simulink model "LFC_3area_fastLoadActor"  (R2021b)
settings: Solver=FixedStepAuto  StartTime=0.0  StopTime=350  FixedStep=0.01  RelTol=1e-3
undefined symbols (not defined in the file or in its folder): sigbuilder_block
libraries: deeplib x3
settings Model: Creator=abc19  LastModifiedBy=abc19
settings SolverCC: AlgebraicLoopSolver=TrustRegion
settings DebuggingCC: SFMachineParentedDataDiag=warning
settings SFSimCC: SimTargetLang=C++

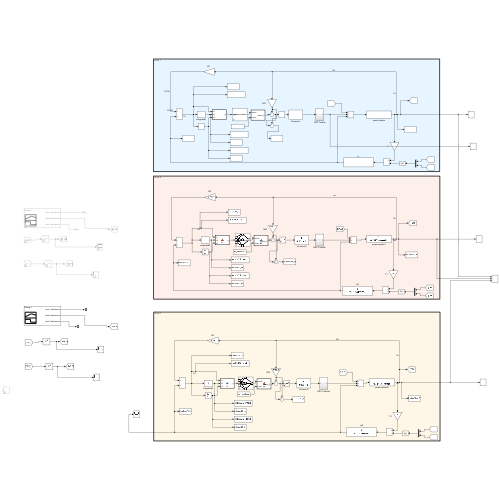
[thumbnail: Simulink's stored preview of the top-level diagram]
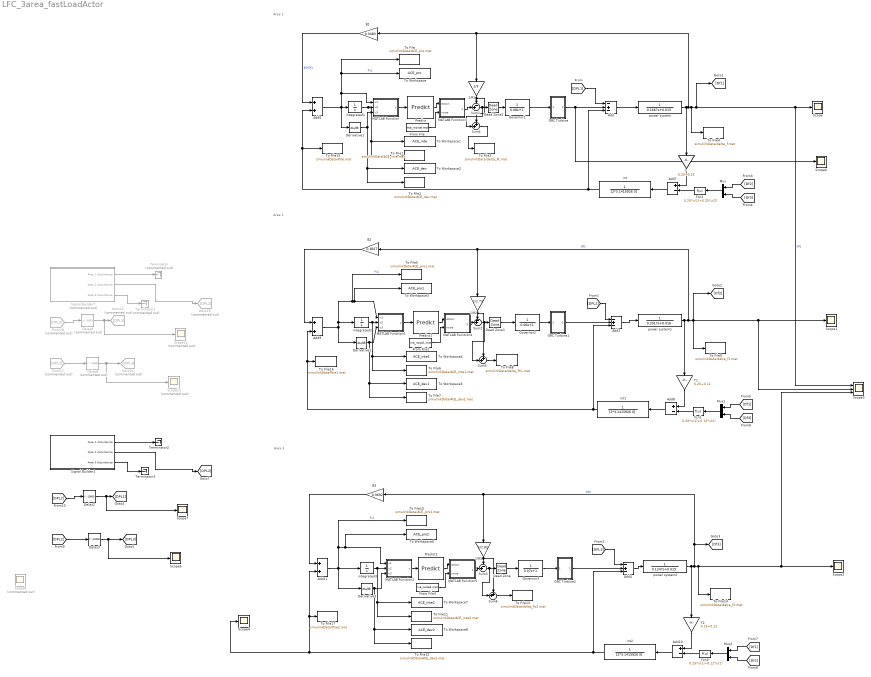
== system LFC_3area_fastLoadActor ==
  note: Area 1
  note: Area 3
  note: Area 2
  1/R1 : Gain  Gain=1/3
  1/R2 : Gain  Gain=1/2.73
  1/R3 : Gain  Gain=1/2.82
  Add : Sum  Inputs=-+-
  Add10 : Sum  Inputs=+-
  Add11 : Sum
  Add2 : Sum  Inputs=-+-
  Add4 : Sum  Inputs=-+-
  Add6 : Sum
  Add7 : Sum  Inputs=+-
  Add8 : Sum  Inputs=+-
  Add9 : Sum
  B1 : Gain  Gain=0.3483
  B2 : Gain  Gain=0.3827
  B3 : Gain  Gain=0.3692
  Dead Zone : DeadZone  LowerValue=-0.00638  UpperValue=0.00638  SaturateOnIntegerOverflow=on
  Dead Zone1 : DeadZone  LowerValue=-0.00659  UpperValue=0.00659  SaturateOnIntegerOverflow=on
  Dead Zone2 : DeadZone  LowerValue=-0.006  UpperValue=0.006  SaturateOnIntegerOverflow=on
  Delay2 : Delay  DelayLength=10000  InitialCondition=0
  Delay3 : Delay  DelayLength=20000  InitialCondition=0
  Delay8 : Delay  Commented=on  DelayLength=5000  InitialCondition=0
  Delay9 : Delay  Commented=on  DelayLength=10000  InitialCondition=0
  Derivative1 : Derivative
  Derivative2 : Derivative
  Derivative3 : Derivative
  Fcn1 : Fcn  Expr=0.20*u(1)+0.12*u(2)
  Fcn2 : Fcn  Expr=0.20*u(1)+0.25*u(2)
  Fcn3 : Fcn  Expr=0.25*u(1)+0.12*u(2)
  From File : FromFile  FileName=ma_noise.mat  SampleTime=0
  From File1 : FromFile  FileName=ma_noise1.mat  SampleTime=0
  From File3 : FromFile  FileName=ma_noise2.mat  SampleTime=0
  From17 : From  Commented=on  GotoTag=DPL2
  From18 : From  Commented=on  GotoTag=DPL2
  GRC Turbine : Subsystem
  GRC Turbine1 : Subsystem
  GRC Turbine2 : Subsystem
  Goto22 : Goto  Commented=on  GotoTag=DPL1
  Goto23 : Goto  Commented=on  GotoTag=DPL3
  Goto25 : Goto  Commented=on  GotoTag=DPL2
  Governor1 : TransferFcn  Denominator=[0.08 1]
  Governor2 : TransferFcn  Denominator=[0.06 1]
  Governor3 : TransferFcn  Denominator=[0.07 1]
  MATLAB Function : MATLAB Function  TreatAsAtomicUnit=on  SystemSampleTime=0.01
  MATLAB Function1 : MATLAB Function  TreatAsAtomicUnit=on  SystemSampleTime=0.01
  MATLAB Function2 : MATLAB Function  TreatAsAtomicUnit=on  SystemSampleTime=0.01
  MATLAB Function3 : MATLAB Function  TreatAsAtomicUnit=on  SystemSampleTime=0.01
  MATLAB Function4 : MATLAB Function  TreatAsAtomicUnit=on  SystemSampleTime=0.01
  MATLAB Function5 : MATLAB Function  TreatAsAtomicUnit=on  SystemSampleTime=0.01
  Mux : Mux  Inputs=2
  Mux1 : Mux  Inputs=2
  Mux2 : Mux  Inputs=2
  Predict : deeplib/Predict  Network=Network from MAT-file  NetworkFunction=squeezenet  NetworkFilePath=aaa.mat  MiniBatchSize=1  InputDataFormats={ '', '' }  Predictions=on  Activations={}  ForceInterpretedSim=off  EnableDLNetwork=on
      settings: SourceProductBaseCode=NN
  Predict1 : deeplib/Predict  Network=Network from MAT-file  NetworkFunction=squeezenet  NetworkFilePath=bbb.mat  MiniBatchSize=1  InputDataFormats={ '', '' }  Predictions=on  Activations={}  ForceInterpretedSim=off  EnableDLNetwork=on
      settings: SourceProductBaseCode=NN
  Predict2 : deeplib/Predict  Network=Network from MAT-file  NetworkFunction=squeezenet  NetworkFilePath=ccc.mat  MiniBatchSize=1  InputDataFormats={ '', '' }  Predictions=on  Activations={}  ForceInterpretedSim=off  EnableDLNetwork=on
      settings: SourceProductBaseCode=NN
  Scope{,1..2,4..7} (7 alike) : Scope
  Scope13 : Scope  Commented=on
  Scope14 : Scope  Commented=on
  Scope3 : Scope  NumInputPorts=3
  Scope8 : Scope  Commented=on
  Signal Builder1 : Subsystem  Tag=STV Subsys  LoadFcn=sigbuilder_block('load');  StartFcn=sigbuilder_block('start');  StopFcn=sigbuilder_block('stop');  ClipboardFcn=sigbuilder_block('clipboard');  mask(Sigbuilder block){tuvar=[0:10]}
      mask help: Simulink:masks:SigbuilderBlock_MD
      mask init:
      | if ~strcmp(get_param(bdroot(gcbh),'SimulationStatus'),'stopped') tuvar = sigbuilder_block('maskInit'); end
      settings: CopyFcn=sigbuilder_block('copy');  DeleteFcn=sigbuilder_block('delete');  ModelCloseFcn=sigbuilder_block('modelClose');  PreSaveFcn=sigbuilder_block('preSave');  PauseFcn=sigbuilder_block('pause');  ContinueFcn=sigbuilder_block('continue');  NameChangeFcn=sigbuilder_block('namechange');  OpenFcn=sigbuilder_block('open',[259.2 170.4 1141.2 408.6 ]);  CloseFcn=sigbuilder_block('close');
      mask Display: plot(0, 0, 100, 100,[2, 2, 32, 32, 2], [68, 8, 8, 68, 68],[32, 2], [38, 38], [32, 19, 2],[53, 60, 44], [32, 17, 17, 2],[16, 16, 31, 31]);txt = getActiveGroup(gcbh);text(2, 100, txt,'verticalAlignment', 'top');
  Signal Builder7 : Subsystem  Tag=STV Subsys  Commented=on  LoadFcn=sigbuilder_block('load');  StartFcn=sigbuilder_block('start');  StopFcn=sigbuilder_block('stop');  ClipboardFcn=sigbuilder_block('clipboard');  mask(Sigbuilder block){tuvar=[0:10]}
      mask help: Simulink:masks:SigbuilderBlock_MD
      mask init:
      | if ~strcmp(get_param(bdroot(gcbh),'SimulationStatus'),'stopped') tuvar = sigbuilder_block('maskInit'); end
      settings: CopyFcn=sigbuilder_block('copy');  DeleteFcn=sigbuilder_block('delete');  ModelCloseFcn=sigbuilder_block('modelClose');  PreSaveFcn=sigbuilder_block('preSave');  PauseFcn=sigbuilder_block('pause');  ContinueFcn=sigbuilder_block('continue');  NameChangeFcn=sigbuilder_block('namechange');  OpenFcn=sigbuilder_block('open',[69 85.8 1141.2 485.4 ]);  CloseFcn=sigbuilder_block('close');
      mask Display: plot(0, 0, 100, 100,[2, 2, 32, 32, 2], [68, 8, 8, 68, 68],[32, 2], [38, 38], [32, 19, 2],[53, 60, 44], [32, 17, 17, 2],[16, 16, 31, 31]);txt = getActiveGroup(gcbh);text(2, 100, txt,'verticalAlignment', 'top');
  Sum1 : Sum  Inputs=-+|
  Sum2 : Sum  Inputs=-+|
  Sum3 : Sum  Inputs=-+|
  Sum4 : Sum  Inputs=++|
  Sum5 : Sum  Inputs=++|
  Sum6 : Sum  Inputs=++|
  T : Gain  Gain=0.20+0.25
  T1 : Gain  Gain=0.20+0.12
  T2 : Gain  Gain=0.25+0.12
  Terminator : Terminator  Commented=on
  Terminator1 : Terminator  Commented=on
  Terminator2 : Terminator
  Terminator3 : Terminator
  To File : ToFile  Filename=simulinkData/ACE_pro.mat  SampleTime=0.01
  To File1 : ToFile  Filename=simulinkData/ACE_inte.mat  SampleTime=0.01
  To File10 : ToFile  Filename=simulinkData/ACE_pro2.mat  SampleTime=0.01
  To File11 : ToFile  Filename=simulinkData/ACE_inte2.mat  SampleTime=0.01
  To File12 : ToFile  Filename=simulinkData/ACE_dev2.mat  SampleTime=0.01
  To File13 : ToFile  Filename=simulinkData/delta_Pc2.mat  SampleTime=0.01
  To File14 : ToFile  Filename=simulinkData/delta_f2.mat  SampleTime=0.01
  To File15 : ToFile  Filename=simulinkData/Ptie.mat  SampleTime=0.01
  To File16 : ToFile  Filename=simulinkData/Ptie1.mat  SampleTime=0.01
  To File17 : ToFile  Filename=simulinkData/Ptie2.mat  SampleTime=0.01
  To File2 : ToFile  Filename=simulinkData/ACE_dev.mat  SampleTime=0.01
  To File3 : ToFile  Filename=simulinkData/delta_Pc.mat  SampleTime=0.01
  To File4 : ToFile  Filename=simulinkData/delta_f.mat  SampleTime=0.01
  To File5 : ToFile  Filename=simulinkData/ACE_pro1.mat  SampleTime=0.01
  To File6 : ToFile  Filename=simulinkData/ACE_inte1.mat  SampleTime=0.01
  To File7 : ToFile  Filename=simulinkData/ACE_dev1.mat  SampleTime=0.01
  To File8 : ToFile  Filename=simulinkData/delta_Pc1.mat  SampleTime=0.01
  To File9 : ToFile  Filename=simulinkData/delta_f1.mat  SampleTime=0.01
  To Workspace : ToWorkspace  VariableName=ACE_pro  SaveFormat=Timeseries  SampleTime=0.01
  To Workspace1 : ToWorkspace  VariableName=ACE_inte  SaveFormat=Timeseries  SampleTime=0.01
  To Workspace2 : ToWorkspace  VariableName=ACE_dev  SaveFormat=Timeseries  SampleTime=0.01
  To Workspace3 : ToWorkspace  VariableName=ACE_pro1  SaveFormat=Timeseries  SampleTime=0.01
  To Workspace4 : ToWorkspace  VariableName=ACE_inte1  SaveFormat=Timeseries  SampleTime=0.01
  To Workspace5 : ToWorkspace  VariableName=ACE_dev1  SaveFormat=Timeseries  SampleTime=0.01
  To Workspace6 : ToWorkspace  VariableName=ACE_pro2  SaveFormat=Timeseries  SampleTime=0.01
  To Workspace7 : ToWorkspace  VariableName=ACE_inte2  SaveFormat=Timeseries  SampleTime=0.01
  To Workspace8 : ToWorkspace  VariableName=ACE_dev2  SaveFormat=Timeseries  SampleTime=0.01
  int : TransferFcn  Denominator=[2*3.1415926 0]
  int1 : TransferFcn  Denominator=[2*3.1415926 0]
  int2 : TransferFcn  Denominator=[2*3.1415926 0]
  integrated1 : TransferFcn  Denominator=[1 0]
  integrated2 : TransferFcn  Denominator=[1 0]
  integrated3 : TransferFcn  Denominator=[1 0]
  power system : TransferFcn  Denominator=[0.1667 0.015]
  power system1 : TransferFcn  Denominator=[0.2017 0.016]
  power system2 : TransferFcn  Denominator=[0.1247 0.015]
  wires:
  [DPL1] -> Add/1
  power system/1 -> To File4/1, [Df1], Scope3/1, Scope/1, B1/1, 1/R1/1, T/1  "Df1"
  GRC Turbine/1(Out1) -> Scope6/1, Add/2
  Add/1 -> power system/1
  B1/1 -> Add6/1  "B1*Df1"
  1/R1/1 -> Sum4/1, Sum1/1
  Governor1/1 -> GRC Turbine/1(In1)
  Sum1/1 -> Sum4/2, Dead Zone2/1
  Derivative1/1 -> To File2/1, To Workspace2/1, MATLAB Function/3(u3)
  integrated1/1 -> To File1/1, To Workspace1/1, MATLAB Function/2(u2)
  Add2/1 -> power system1/1
  Sum2/1 -> Sum5/2, Dead Zone1/1
  1/R2/1 -> Sum5/1, Sum2/1
  Governor2/1 -> GRC Turbine1/1(In1)
  GRC Turbine1/1(Out1) -> Add2/2
  [DPL2] -> Add2/1
  Add4/1 -> power system2/1
  Sum3/1 -> Sum6/2, Dead Zone/1
  1/R3/1 -> Sum6/1, Sum3/1
  Governor3/1 -> GRC Turbine2/1(In1)
  GRC Turbine2/1(Out1) -> Add4/2
  [DPL3] -> Add4/1
  int/1 -> Add6/2, To File15/1, Add/3
  Add6/1 -> Derivative1/1, To Workspace/1, To File/1, MATLAB Function/1(u1), integrated1/1  "Pc1"
  Add7/1 -> int/1
  T/1 -> Add7/1
  Fcn2/1 -> Add7/2
  Mux/1 -> Fcn2/1
  [Df2] -> Mux/1
  [Df3] -> Mux/2
  [Df1] -> Mux1/1
  [Df3] -> Mux1/2
  Mux1/1 -> Fcn1/1
  power system1/1 -> To File9/1, [Df2], Scope3/2, Scope1/1, B2/1, 1/R2/1, T1/1  "Df2"
  T1/1 -> Add8/1
  int1/1 -> To File16/1, Add9/2, Add2/3
  Add8/1 -> int1/1
  Fcn1/1 -> Add8/2
  B2/1 -> Add9/1
  [Df1] -> Mux2/1
  [Df2] -> Mux2/2
  Mux2/1 -> Fcn3/1
  power system2/1 -> [Df3], B3/1, 1/R3/1, To File14/1, Scope3/3, Scope2/1, T2/1  "Df3"
  T2/1 -> Add10/1
  int2/1 -> Scope4/1, To File17/1, Add11/2, Add4/3
  Add10/1 -> int2/1
  Fcn3/1 -> Add10/2
  B3/1 -> Add11/1
  Dead Zone/1 -> Governor3/1
  Dead Zone1/1 -> Governor2/1
  Dead Zone2/1 -> Governor1/1
  MATLAB Function/1(y) -> Predict/1
  MATLAB Function3/1(action_2) -> Sum1/2
  Predict/1 -> MATLAB Function3/1(action)
  Predict1/1 -> MATLAB Function4/1(action)
  integrated2/1 -> To File6/1, To Workspace4/1, MATLAB Function1/2(u2)
  MATLAB Function4/1(action_2) -> Sum2/2
  Derivative2/1 -> MATLAB Function1/3(u3), To File7/1, To Workspace5/1
  MATLAB Function1/1(y) -> Predict1/1
  Add9/1 -> Derivative2/1, MATLAB Function1/1(u1), To Workspace3/1, To File5/1, integrated2/1  "Pc1"
  Predict2/1 -> MATLAB Function5/1(action)
  integrated3/1 -> MATLAB Function2/2(u2), To File11/1, To Workspace7/1
  MATLAB Function5/1(action_2) -> Sum3/2
  Derivative3/1 -> MATLAB Function2/3(u3), To File12/1, To Workspace8/1
  MATLAB Function2/1(y) -> Predict2/1
  Add11/1 -> To File10/1, MATLAB Function2/1(u1), To Workspace6/1, Derivative3/1, integrated3/1  "Pc1"
  Sum4/1 -> To File3/1
  Sum5/1 -> To File8/1
  Sum6/1 -> To File13/1
  Signal Builder7/2(Area 2 disturbance) -> Goto25/1
  Delay8/1 -> Scope14/1, Goto22/1
  From17/1 -> Delay9/1
  Delay9/1 -> Goto23/1, Scope13/1
  From18/1 -> Delay8/1
  From File/1 -> MATLAB Function3/2(noise)
  From File1/1 -> MATLAB Function4/2(noise)
  From File3/1 -> MATLAB Function5/2(noise)
  Signal Builder7/1(Area 1 disturbance) -> Terminator/1
  Signal Builder7/3(Area 3 disturbance) -> Terminator1/1
  Signal Builder1/3(Area 3 disturbance) -> Terminator3/1
  Delay3/1 -> Scope5/1, [DPL3]
  Signal Builder1/2(Area 2 disturbance) -> [DPL2]
  [DPL2] -> Delay2/1
  [DPL2] -> Delay3/1
  Signal Builder1/1(Area 1 disturbance) -> Terminator2/1
  Delay2/1 -> [DPL1], Scope7/1

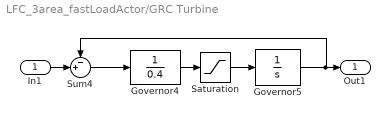
== system LFC_3area_fastLoadActor/GRC Turbine ==
  In1 : Inport
  Governor4 : TransferFcn  Denominator=[0.4]
  Governor5 : TransferFcn  Denominator=[1 0]
  Saturation : Saturate  UpperLimit=0.0017  LowerLimit=-0.0017
  Sum4 : Sum  Inputs=-+|
  Out1 : Outport
  wires:
  Governor5/1 -> Sum4/1, Out1/1
  Governor4/1 -> Saturation/1
  Sum4/1 -> Governor4/1
  Saturation/1 -> Governor5/1
  In1/1 -> Sum4/2

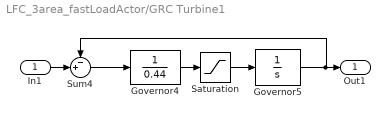
== system LFC_3area_fastLoadActor/GRC Turbine1 ==
  In1 : Inport
  Governor4 : TransferFcn  Denominator=[0.44]
  Governor5 : TransferFcn  Denominator=[1 0]
  Saturation : Saturate  UpperLimit=0.0017  LowerLimit=-0.0017
  Sum4 : Sum  Inputs=-+|
  Out1 : Outport
  wires:
  Governor5/1 -> Sum4/1, Out1/1
  Governor4/1 -> Saturation/1
  Sum4/1 -> Governor4/1
  Saturation/1 -> Governor5/1
  In1/1 -> Sum4/2

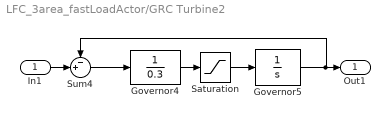
== system LFC_3area_fastLoadActor/GRC Turbine2 ==
  In1 : Inport
  Governor4 : TransferFcn  Denominator=[0.3]
  Governor5 : TransferFcn  Denominator=[1 0]
  Saturation : Saturate  UpperLimit=0.0017  LowerLimit=-0.0017
  Sum4 : Sum  Inputs=-+|
  Out1 : Outport
  wires:
  Governor5/1 -> Sum4/1, Out1/1
  Governor4/1 -> Saturation/1
  Sum4/1 -> Governor4/1
  Saturation/1 -> Governor5/1
  In1/1 -> Sum4/2

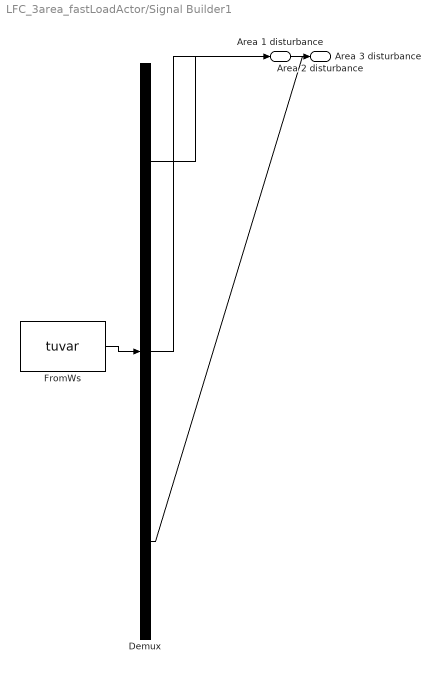
== system LFC_3area_fastLoadActor/Signal Builder1 ==
  Demux : Demux  Tag=STV Demux  Outputs=3
      settings: DisplayOption=none
  FromWs : FromWorkspace  Tag=STV FromWs  VariableName=tuvar
      SigBuilderData=|
      | common.afterFinalStr = 'Extrapolate'
      | common.sampleTime = 0
      | dataSet.timeRange = [0 400]
      | dataSet.name = 'Group 1'
      | sbobj.Groups.Name = 'Group 1'
      | sbobj.Groups.Signals(1).Name = 'Area 1 disturbance'
      | sbobj.Groups.Signals(1).XData = [0 30 30 60 60 400]
      | sbobj.Groups.Signals(1).YData = [0.01 0.01 -0.01 -0.01 0.01 0.01]
      | sbobj.Groups.Signals(2).Name = 'Area 2 disturbance'
      | sbobj.Groups.Signals(2).XData = [0 50 50 100 100 400]
      | sbobj.Groups.Signals(2).YData = [0 0 0.01 0.01 0 0]
      | sbobj.Groups.Signals(3).Name = 'Area 3 disturbance'
      | sbobj.Groups.Signals(3).XData = [0 400]
      | sbobj.Groups.Signals(3).YData = [0 0]
      | sbobj.Groups.TimeRange = [0 400]
  Area 1 disturbance : Outport  Tag=STV Outport
  Area 2 disturbance : Outport  Tag=STV Outport  Port=2
  Area 3 disturbance : Outport  Tag=STV Outport  Port=3
  wires:
  Demux/1 -> Area 1 disturbance/1
  FromWs/1 -> Demux/1
  Demux/2 -> Area 2 disturbance/1
  Demux/3 -> Area 3 disturbance/1

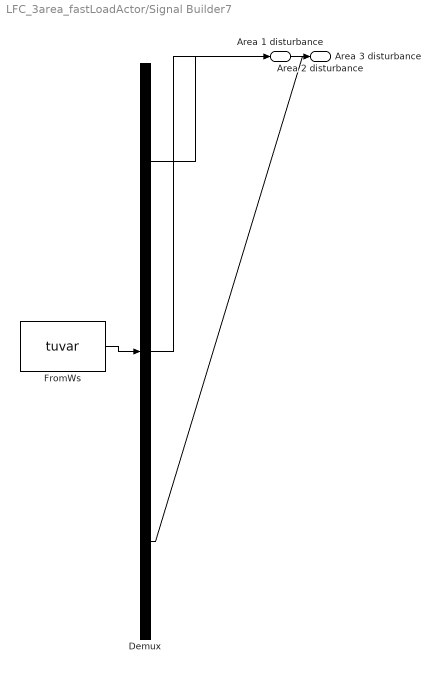
== system LFC_3area_fastLoadActor/Signal Builder7 ==
  Demux : Demux  Tag=STV Demux  Outputs=3
      settings: DisplayOption=none
  FromWs : FromWorkspace  Tag=STV FromWs  VariableName=tuvar
      SigBuilderData=|
      | common.afterFinalStr = 'Extrapolate'
      | common.sampleTime = 0
      | dataSet.timeRange = [0 400]
      | dataSet.name = 'Group 1'
      | sbobj.Groups.Name = 'Group 1'
      | sbobj.Groups.Signals(1).Name = 'Area 1 disturbance'
      | sbobj.Groups.Signals(1).XData = [0 30 30 60 60 400]
      | sbobj.Groups.Signals(1).YData = [0.01 0.01 -0.01 -0.01 0.01 0.01]
      | sbobj.Groups.Signals(2).Name = 'Area 2 disturbance'
      | sbobj.Groups.Signals(2).XData = [0 50 50 200 200 400]
      | sbobj.Groups.Signals(2).YData = [0 0 0.01 0.01 0 0]
      | sbobj.Groups.Signals(3).Name = 'Area 3 disturbance'
      | sbobj.Groups.Signals(3).XData = [0 400]
      | sbobj.Groups.Signals(3).YData = [0 0]
      | sbobj.Groups.TimeRange = [0 400]
  Area 1 disturbance : Outport  Tag=STV Outport
  Area 2 disturbance : Outport  Tag=STV Outport  Port=2
  Area 3 disturbance : Outport  Tag=STV Outport  Port=3
  wires:
  Demux/3 -> Area 3 disturbance/1
  Demux/2 -> Area 2 disturbance/1
  FromWs/1 -> Demux/1
  Demux/1 -> Area 1 disturbance/1

== matlab function LFC_3area_fastLoadActor/MATLAB Function1 ==
  settings: updateMethod=DISCRETE  sampleTime=0.01
  data: u1 input; y output; u2 input; u3 input
function y = fcn(u1, u2 ,u3)
num =2;
% net = coder.loadDeepLearningNetwork('bbb.mat');
statemax = [[0.0290, 0.0722, 0.0209]
                     [0.0301, 0.0932, 0.0190]
                     [0.0364, 0.0759, 0.0296]];
statemin = [[-0.0291, -0.0948, -0.0209]
                     [-0.0301, -0.1150, -0.0190]
                     [-0.0363, -0.1110, -0.0296]];
actionmax = [0.0931, 0.0994, 0.1090];
actionmin = [-0.0708, -0.0810, -0.0855];
y1 = (u1-statemin(num ,1))/(statemax(num, 1) - statemin(num, 1));
y2 = (u2-statemin(num ,2))/(statemax(num, 2) - statemin(num, 2));
y3 = (u3-statemin(num ,3))/(statemax(num, 3) - statemin(num, 3));
y =[y1, y2,y3];
% action = predict(net, [u1, u2, u3]);
% action = action*(actionmax(num)-actionmin(num)) + actionmin(num);
% y = double(action);

== matlab function LFC_3area_fastLoadActor/MATLAB Function ==
  settings: updateMethod=DISCRETE  sampleTime=0.01
  data: u1 input; y output; u2 input; u3 input
function y = fcn(u1, u2 ,u3)
num =1;
% net = coder.loadDeepLearningNetwork('bbb.mat');
statemax = [[0.0290, 0.0722, 0.0209]
                     [0.0301, 0.0932, 0.0190]
                     [0.0364, 0.0759, 0.0296]];
statemin = [[-0.0291, -0.0948, -0.0209]
                     [-0.0301, -0.1150, -0.0190]
                     [-0.0363, -0.1110, -0.0296]];
actionmax = [0.0931, 0.0994, 0.1090];
actionmin = [-0.0708, -0.0810, -0.0855];

y1 = (u1-statemin(num ,1))/(statemax(num, 1) - statemin(num, 1));
y2 = (u2-statemin(num ,2))/(statemax(num, 2) - statemin(num, 2));
y3 = (u3-statemin(num ,3))/(statemax(num, 3) - statemin(num, 3));
y =[y1, y2,y3];
% action = predict(net, [u1, u2, u3]);
% action = action*(actionmax(num)-actionmin(num)) + actionmin(num);
% y = double(action);

== matlab function LFC_3area_fastLoadActor/MATLAB Function2 ==
  settings: updateMethod=DISCRETE  sampleTime=0.01
  data: u1 input; y output; u2 input; u3 input
function y = fcn(u1, u2 ,u3)
num =3;
% net = coder.loadDeepLearningNetwork('bbb.mat');
statemax = [[0.0290, 0.0722, 0.0209]
                     [0.0301, 0.0932, 0.0190]
                     [0.0364, 0.0759, 0.0296]];
statemin = [[-0.0291, -0.0948, -0.0209]
                     [-0.0301, -0.1150, -0.0190]
                     [-0.0363, -0.1110, -0.0296]];
actionmax = [0.0931, 0.0994, 0.1090];
actionmin = [-0.0708, -0.0810, -0.0855];

y1 = (u1-statemin(num ,1))/(statemax(num, 1) - statemin(num, 1));
y2 = (u2-statemin(num ,2))/(statemax(num, 2) - statemin(num, 2));
y3 = (u3-statemin(num ,3))/(statemax(num, 3) - statemin(num, 3));
y =[y1, y2,y3];
% action = predict(net, [u1, u2, u3]);
% action = action*(actionmax(num)-actionmin(num)) + actionmin(num);
% y = double(action);

== matlab function LFC_3area_fastLoadActor/MATLAB Function3 ==
  settings: updateMethod=DISCRETE  sampleTime=0.01
  data: action input; action_2 output; noise input
function action_2= fcn(action, noise)
num =1;
noise =1 ;
statemax = [[0.0290, 0.0722, 0.0209]
                     [0.0301, 0.0932, 0.0190]
                     [0.0364, 0.0759, 0.0296]];
statemin = [[-0.0291, -0.0948, -0.0209]
                     [-0.0301, -0.1150, -0.0190]
                     [-0.0363, -0.1110, -0.0296]];
actionmax = [0.0931, 0.0994, 0.1090];
actionmin = [-0.0708, -0.0810, -0.0855];

action_2 = double(noise * (action*(actionmax(num)-actionmin(num)) + actionmin(num)));

== matlab function LFC_3area_fastLoadActor/MATLAB Function4 ==
  settings: updateMethod=DISCRETE  sampleTime=0.01
  data: action input; action_2 output; noise input
function action_2= fcn(action, noise)
num =2;
noise = 1;
statemax = [[0.0290, 0.0722, 0.0209]
                     [0.0301, 0.0932, 0.0190]
                     [0.0364, 0.0759, 0.0296]];
statemin = [[-0.0291, -0.0948, -0.0209]
                     [-0.0301, -0.1150, -0.0190]
                     [-0.0363, -0.1110, -0.0296]];
actionmax = [0.0931, 0.0994, 0.1090];
actionmin = [-0.0708, -0.0810, -0.0855];

action_2 = double(noise*(action*(actionmax(num)-actionmin(num)) + actionmin(num)));

== matlab function LFC_3area_fastLoadActor/MATLAB Function5 ==
  settings: updateMethod=DISCRETE  sampleTime=0.01
  data: action input; action_2 output; noise input
function action_2= fcn(action, noise)
num =3;
noise = 1;
statemax = [[0.0290, 0.0722, 0.0209]
                     [0.0301, 0.0932, 0.0190]
                     [0.0364, 0.0759, 0.0296]];
statemin = [[-0.0291, -0.0948, -0.0209]
                     [-0.0301, -0.1150, -0.0190]
                     [-0.0363, -0.1110, -0.0296]];
actionmax = [0.0931, 0.0994, 0.1090];
actionmin = [-0.0708, -0.0810, -0.0855];
action_2 = double(noise *(action*(actionmax(num)-actionmin(num)) + actionmin(num)));
